simulink model "PID"  (R2022b)
settings: Solver=VariableStepAuto  StartTime=0.0  StopTime=100.0  RelTol=1e-3
settings Model: Creator=huber  LastModifiedBy=huber

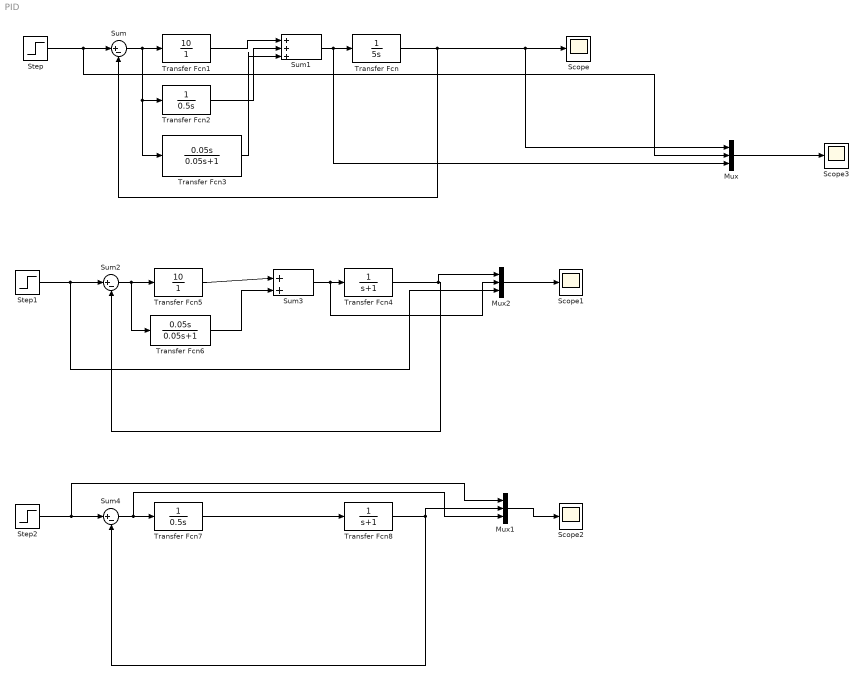
== system PID ==
  Mux : Mux  Inputs=3
  Mux1 : Mux  Inputs=3
  Mux2 : Mux  Inputs=3
  Scope{,1..3} (4 alike) : Scope
  Step : Step  Time=0.1  Before=0.5  After=0.8  SampleTime=0
  Step1 : Step  Time=0.1  Before=0.5  After=0.8  SampleTime=0
  Step2 : Step  Time=0.1  Before=0.5  After=0.8  SampleTime=0
  Sum : Sum  Inputs=|+-
  Sum1 : Sum  Inputs=|+++
  Sum2 : Sum  Inputs=|+-
  Sum3 : Sum  Inputs=|++
  Sum4 : Sum  Inputs=|+-
  Transfer Fcn : TransferFcn  Denominator=[ 5 0]
  Transfer Fcn1 : TransferFcn  Numerator=[10]  Denominator=[0 1]
  Transfer Fcn2 : TransferFcn  Denominator=[0.5 0]
  Transfer Fcn3 : TransferFcn  Numerator=[0.05 0]  Denominator=[0.05 1]
  Transfer Fcn4 : TransferFcn  Denominator=[1 1]
  Transfer Fcn5 : TransferFcn  Numerator=[10]  Denominator=[0 1]
  Transfer Fcn6 : TransferFcn  Numerator=[0.05 0]  Denominator=[0.05 1]
  Transfer Fcn7 : TransferFcn  Denominator=[0.5 0]
  Transfer Fcn8 : TransferFcn  Denominator=[1 1]
  wires:
  Step/1 -> Mux/2, Sum/1
  Sum/1 -> Transfer Fcn3/1, Transfer Fcn2/1, Transfer Fcn1/1
  Transfer Fcn1/1 -> Sum1/1
  Sum1/1 -> Mux/3, Transfer Fcn/1
  Transfer Fcn2/1 -> Sum1/2
  Transfer Fcn3/1 -> Sum1/3
  Sum3/1 -> Mux2/2, Transfer Fcn4/1
  Sum2/1 -> Transfer Fcn6/1, Transfer Fcn5/1
  Transfer Fcn4/1 -> Mux2/1, Sum2/2
  Step1/1 -> Mux2/3, Sum2/1
  Transfer Fcn5/1 -> Sum3/1
  Sum4/1 -> Transfer Fcn7/1, Mux1/3
  Transfer Fcn8/1 -> Mux1/2, Sum4/2
  Step2/1 -> Mux1/1, Sum4/1
  Transfer Fcn7/1 -> Transfer Fcn8/1
  Mux/1 -> Scope3/1
  Transfer Fcn/1 -> Mux/1, Scope/1, Sum/2
  Mux1/1 -> Scope2/1
  Mux2/1 -> Scope1/1
  Transfer Fcn6/1 -> Sum3/2
